simulink model "ctrl_clean_room_sim"  (R2015b)
settings: Solver=ode1  StartTime=0.0  StopTime=30  FixedStep=0.002  RelTol=1e-3
values from neighbouring files (symbols this model uses):
  K = place(A', C', p)'    [high_gain_pole_placement.m]    (also in tvlqr_feedback_trajectory.m = zeros(length(t), m, n); tvlqri_feedback_trajectory.m = zeros(length(t), m, n); weird_observer_pole_placement.m)
  lamb = [0  0  0  0  0; 0  0  0  0  0]    [dyn_ext_eps_static_meas.mat]    (also in extend_static_trajectory.m = repmat(lamb, samples, 1); high_gain_obs_test_meas_using_obs_for_contr.mat = [0 1.24633399283e-14 3.94751216865e-13 2.99125768707e-12 1.2; high_gain_obs_test_meas_using_obs_for_contr_2.mat = [0 0 0 0 0 0 0 0 0 0 0 0 ... (30000 elements, 6000x5)]; high_gain_obs_test_meas_using_obs_for_contr_3.mat = [0 0 0 0 0 0 0 0 0 0 0 0 ... (30000 elements, 6000x5)])
  logts = log.time    [ctr_sim_prepare_ws.m]
  logvals = zeros(numel(logts), n_signals)    [ctr_sim_prepare_ws.m]
  phi = [0  0  0; 0  0  0]    [dyn_ext_eps_static_meas.mat]    (also in extend_static_trajectory.m = repmat(phi, samples, 1); high_gain_obs_test_meas_using_obs_for_contr.mat = [1.104382406e-14 3.36532550257e-09 2.6875311489e-08 9.054493; high_gain_obs_test_meas_using_obs_for_contr_2.mat = [0 0 0 0 0 0 0 0 0 0 0 0 ... (18000 elements, 6000x3)]; high_gain_obs_test_meas_using_obs_for_contr_3.mat = [0 0 0 0 0 0 0 0 0 0 0 0 ... (18000 elements, 6000x3)])
  vb = [3.51031402612 3.51031402612]    [dyn_ext_eps_static_meas.mat]    (also in extend_static_trajectory.m = repmat(vb, samples, 1); high_gain_obs_test_meas_using_obs_for_contr.mat = [3.03305943788 3.03299005654 3.03292056635 3.03285098117 3.0; high_gain_obs_test_meas_using_obs_for_contr_2.mat = [2.46662433384 2.46662437608 2.46662467016 2.46662546356 2.4; high_gain_obs_test_meas_using_obs_for_contr_3.mat = [2.46662433384 2.46662437608 2.46662467016 2.46662546356 2.4)
  vf = [3.51031402612 3.51031402612]    [dyn_ext_eps_static_meas.mat]    (also in extend_static_trajectory.m = repmat(vf, samples, 1); high_gain_obs_test_meas_using_obs_for_contr.mat = [3.03305943788 3.03312882088 3.03319832259 3.03326793896 3.0; high_gain_obs_test_meas_using_obs_for_contr_2.mat = [2.46662433384 2.46662437608 2.46662467016 2.46662546356 2.4; high_gain_obs_test_meas_using_obs_for_contr_3.mat = [2.46662433384 2.46662437608 2.46662467016 2.46662546356 2.4)
undefined symbols (not defined in the file or in its folder): qc_get_step_size, R
libraries: simulink_extras x7, quarc_library x2, simulink x1
settings Model: Creator=Robert  LastModifiedBy=Robert

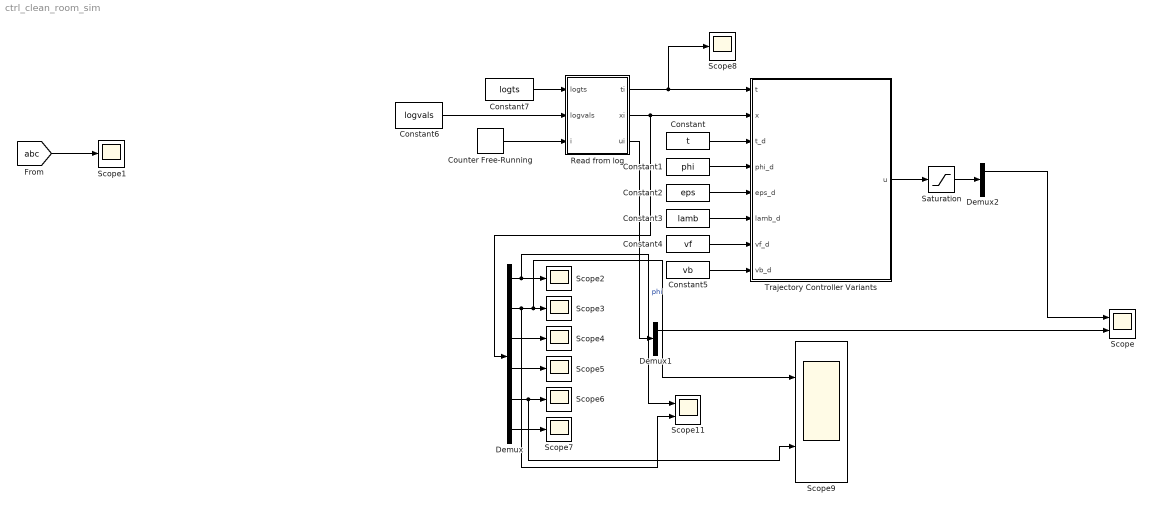
== system ctrl_clean_room_sim ==
  Constant : Constant  Value=t
  Constant1 : Constant  Value=phi
  Constant2 : Constant  Value=eps
  Constant3 : Constant  Value=lamb
  Constant4 : Constant  Value=vf
  Constant5 : Constant  Value=vb
  Constant6 : Constant  Value=logvals
  Constant7 : Constant  Value=logts
  Counter Free-Running : simulink/Sources/Counter Free-Running  NumBits=32  tsamp=-1
  Demux : Demux  Outputs=6
  Demux1 : Demux  Outputs=2
  Demux2 : Demux  Outputs=2
  Read from log : MATLAB Function  TreatAsAtomicUnit=on
  Saturation : Saturate  UpperLimit=5  LowerLimit=-5
  Scope : Scope  NumInputPorts=2
  Scope{1..8} (8 alike) : Scope
  Scope11 : Scope  NumInputPorts=2
  Scope9 : Scope  NumInputPorts=2
  Trajectory Controller Variants : Subsystem  Variant=on  OverrideUsingVariant=StateFeedback
  wires:
  Constant/1 -> Trajectory Controller Variants/3(t_d)
  Constant3/1 -> Trajectory Controller Variants/6(lamb_d)
  Constant2/1 -> Trajectory Controller Variants/5(eps_d)
  Constant1/1 -> Trajectory Controller Variants/4(phi_d)
  Constant5/1 -> Trajectory Controller Variants/8(vb_d)
  Constant4/1 -> Trajectory Controller Variants/7(vf_d)
  Read from log/2(xi) -> Demux/1, Trajectory Controller Variants/2(x)
  Read from log/1(ti) -> Scope8/1, Trajectory Controller Variants/1(t)
  Counter Free-Running/1 -> Read from log/3(i)
  Constant6/1 -> Read from log/2(logvals)
  Constant7/1 -> Read from log/1(logts)
  Read from log/3(ui) -> Demux1/1
  Trajectory Controller Variants/1(u) -> Saturation/1
  Saturation/1 -> Demux2/1
  Demux/1 -> Scope11/1, Scope2/1  "phi"
  Demux/2 -> Scope11/2, Scope9/1, Scope3/1
  Demux/3 -> Scope4/1
  Demux/4 -> Scope5/1
  Demux/5 -> Scope9/2, Scope6/1
  Demux/6 -> Scope7/1
  Demux2/1 -> Scope/1
  Demux1/1 -> Scope/2
  [abc] -> Scope1/1

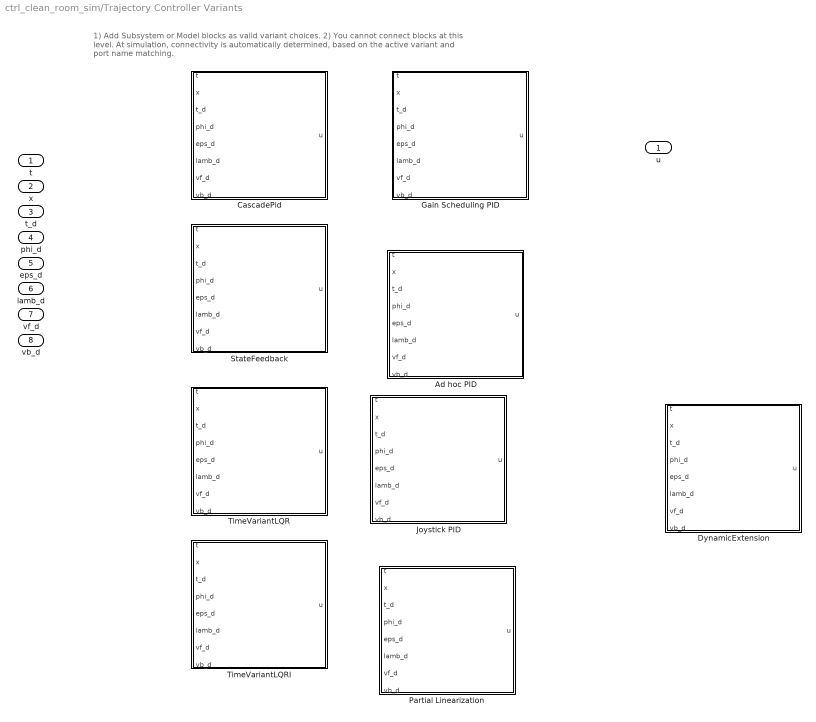
== system ctrl_clean_room_sim/Trajectory Controller Variants ==
  note: 1) Add Subsystem or Model blocks as valid variant choices.
      | 2) You cannot connect blocks at this level. At simulation, connectivity is automatically
      | determined, based on the active variant and port name matching.
  t : Inport
  x : Inport  Port=2  PortDimensions=6
  t_d : Inport  Port=3
  phi_d : Inport  Port=4
  eps_d : Inport  Port=5
  lamb_d : Inport  Port=6
  vf_d : Inport  Port=7
  vb_d : Inport  Port=8
  Ad hoc PID : Subsystem  VariantControl=AdHocPID
  CascadePid : Subsystem  VariantControl=CascadePid
  DynamicExtension : Subsystem  VariantControl=DynamicExtension
  Gain Scheduling PID : Subsystem  VariantControl=GainSchedulingPid
  Joystick PID : Subsystem  VariantControl=JoystickPID
  Partial Linearization : Subsystem  VariantControl=PartialLinearization
  StateFeedback : Subsystem  VariantControl=StateFeedback
  TimeVariantLQR : Subsystem  VariantControl=TimeVariantLQR
  TimeVariantLQRI : Subsystem  VariantControl=TimeVariantLQRI
  u : Outport

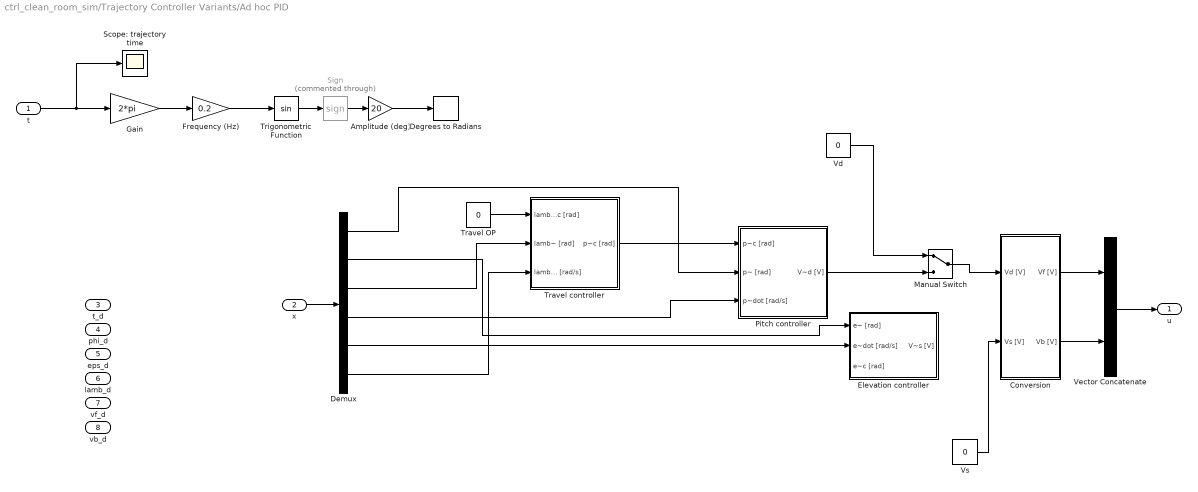
== system ctrl_clean_room_sim/Trajectory Controller Variants/Ad hoc PID ==
  t : Inport
  x : Inport  Port=2
  t_d : Inport  Port=3
  phi_d : Inport  Port=4
  eps_d : Inport  Port=5
  lamb_d : Inport  Port=6
  vf_d : Inport  Port=7
  vb_d : Inport  Port=8
  Amplitude (deg) : Gain  Gain=20
  Conversion : Subsystem
  Degrees to Radians : simulink_extras/Transformations/Degrees to Radians
  Demux : Demux  Outputs=6
  Elevation controller : Subsystem
  Frequency (Hz) : Gain  Gain=0.2
  Gain : Gain  Gain=2*pi
  Manual Switch : ManualSwitch
  Pitch controller : Subsystem
  Scope: trajectory time : Scope
  Sign : Signum  Commented=through
  Travel OP : Constant  Value=0
  Travel controller : Subsystem
  Trigonometric Function : Trigonometry
  Vd : Constant  Value=0
  Vector Concatenate : Concatenate
  Vs : Constant  Value=0
  u : Outport
  wires:
  Conversion/1(Vf [V]) -> Vector Concatenate/1
  Conversion/2(Vb [V]) -> Vector Concatenate/2
  x/1 -> Demux/1
  Demux/1 -> Pitch controller/2(p~ [rad])
  Demux/2 -> Elevation controller/1(e~ [rad])
  Demux/3 -> Travel controller/2(lamb~ [rad])
  Demux/4 -> Pitch controller/3(p~dot [rad/s])
  Demux/5 -> Elevation controller/2(e~dot [rad/s])
  Demux/6 -> Travel controller/3(lamb~dot [rad/s])
  Vector Concatenate/1 -> u/1
  t/1 -> Scope: trajectory time/1, Gain/1
  Gain/1 -> Frequency (Hz)/1
  Frequency (Hz)/1 -> Trigonometric Function/1
  Trigonometric Function/1 -> Sign/1
  Pitch controller/1(V~d [V]) -> Manual Switch/2
  Manual Switch/1 -> Conversion/1(Vd [V])
  Sign/1 -> Amplitude (deg)/1
  Amplitude (deg)/1 -> Degrees to Radians/1
  Travel controller/1(p~c [rad]) -> Pitch controller/1(p~c [rad])
  Travel OP/1 -> Travel controller/1(lamb~c [rad])
  Vd/1 -> Manual Switch/1
  Vs/1 -> Conversion/2(Vs [V])

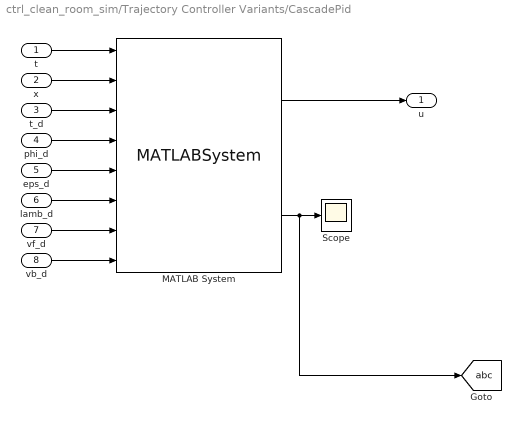
== system ctrl_clean_room_sim/Trajectory Controller Variants/CascadePid ==
  t : Inport
  x : Inport  Port=2
  t_d : Inport  Port=3
  phi_d : Inport  Port=4
  eps_d : Inport  Port=5
  lamb_d : Inport  Port=6
  vf_d : Inport  Port=7
  vb_d : Inport  Port=8
  MATLAB System : MATLABSystem  System=CascadePid  elevation_pid_gains=[15, 3, 7]  travel_pitch_pid_gains=[2.5, 0.5, 3]  pitch_vd_pid_gains=[4, 0.1, 2]  feed_forward=on  SimulateUsing=Code generation
      mask Type: CascadePid
      mask Display:
      | disp('CascadePid');
      | port_label('input',1,'Time');
      | port_label('input',2,'State');
      | port_label('input',3,'Traj Time');
      | port_label('input',4,'Traj Phi');
      | port_label('input',5,'Traj Eps');
      | port_label('input',6,'Traj Lamb');
      | port_label('input',7,'Traj Vf');
      | port_label('input',8,'Traj Vb');
      | port_label('output',1,'Control');
      | port_label('output',2,'Debug');
  Scope : Scope
  u : Outport
  tag scope: abc=global
  wires:
  MATLAB System/1 -> u/1
  vb_d/1 -> MATLAB System/8
  vf_d/1 -> MATLAB System/7
  lamb_d/1 -> MATLAB System/6
  eps_d/1 -> MATLAB System/5
  phi_d/1 -> MATLAB System/4
  t_d/1 -> MATLAB System/3
  x/1 -> MATLAB System/2
  t/1 -> MATLAB System/1
  MATLAB System/2 -> [abc], Scope/1

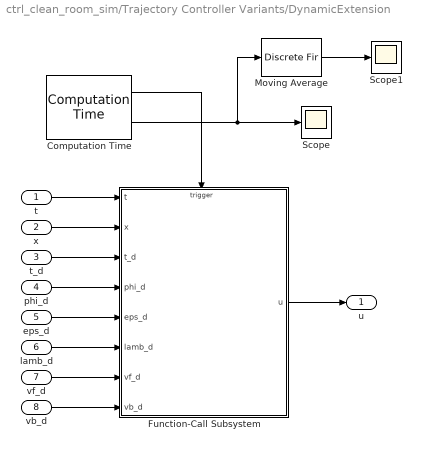
== system ctrl_clean_room_sim/Trajectory Controller Variants/DynamicExtension ==
  t : Inport
  x : Inport  Port=2
  t_d : Inport  Port=3
  phi_d : Inport  Port=4
  eps_d : Inport  Port=5
  lamb_d : Inport  Port=6
  vf_d : Inport  Port=7
  vb_d : Inport  Port=8
  Computation Time : quarc_library/Sources/Time/Computation Time  sample_time=qc_get_step_size  use_model=off
  Function-Call Subsystem : Subsystem  TreatAsAtomicUnit=on
  Moving Average : DiscreteFir  Coefficients=ones(1, 50) / 50
  Scope : Scope
  Scope1 : Scope
  u : Outport
  wires:
  vb_d/1 -> Function-Call Subsystem/8(vb_d)
  vf_d/1 -> Function-Call Subsystem/7(vf_d)
  lamb_d/1 -> Function-Call Subsystem/6(lamb_d)
  eps_d/1 -> Function-Call Subsystem/5(eps_d)
  phi_d/1 -> Function-Call Subsystem/4(phi_d)
  t_d/1 -> Function-Call Subsystem/3(t_d)
  x/1 -> Function-Call Subsystem/2(x)
  t/1 -> Function-Call Subsystem/1(t)
  Function-Call Subsystem/1(u) -> u/1
  Computation Time/1 -> Function-Call Subsystem/Trigger
  Computation Time/2 -> Moving Average/1, Scope/1
  Moving Average/1 -> Scope1/1

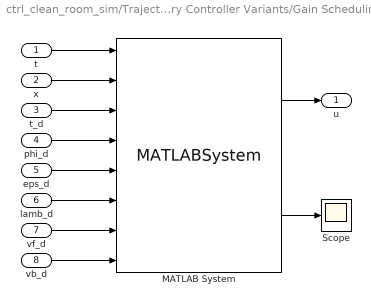
== system ctrl_clean_room_sim/Trajectory Controller Variants/Gain Scheduling PID ==
  t : Inport
  x : Inport  Port=2
  t_d : Inport  Port=3
  phi_d : Inport  Port=4
  eps_d : Inport  Port=5
  lamb_d : Inport  Port=6
  vf_d : Inport  Port=7
  vb_d : Inport  Port=8
  MATLAB System : MATLABSystem  System=GainSchedulingPid  elevation_levels=[ -10, 0, 10, 20 ]  elevation_pid_gains=[15, 3, 7]  travel_pitch_pid_gains=[2.5, 0.1, 3.2; 4, 0.1, 3.5; 4, 0.1, 3.25; 2.5, 0.1, 2.5]  pitch_vd_pid_gains=[ 4, 0.1, 2 ]  feed_forward=on  SimulateUsing=Code generation
      mask Type: GainSchedulingPid
      mask Display:
      | disp('GainSchedulingPid');
      | port_label('input',1,'Time');
      | port_label('input',2,'State');
      | port_label('input',3,'Traj Time');
      | port_label('input',4,'Traj Phi');
      | port_label('input',5,'Traj Eps');
      | port_label('input',6,'Traj Lamb');
      | port_label('input',7,'Traj Vf');
      | port_label('input',8,'Traj Vb');
      | port_label('output',1,'Control');
      | port_label('output',2,'Debug');
  Scope : Scope
  u : Outport
  wires:
  MATLAB System/1 -> u/1
  vb_d/1 -> MATLAB System/8
  vf_d/1 -> MATLAB System/7
  lamb_d/1 -> MATLAB System/6
  eps_d/1 -> MATLAB System/5
  phi_d/1 -> MATLAB System/4
  t_d/1 -> MATLAB System/3
  x/1 -> MATLAB System/2
  t/1 -> MATLAB System/1
  MATLAB System/2 -> Scope/1

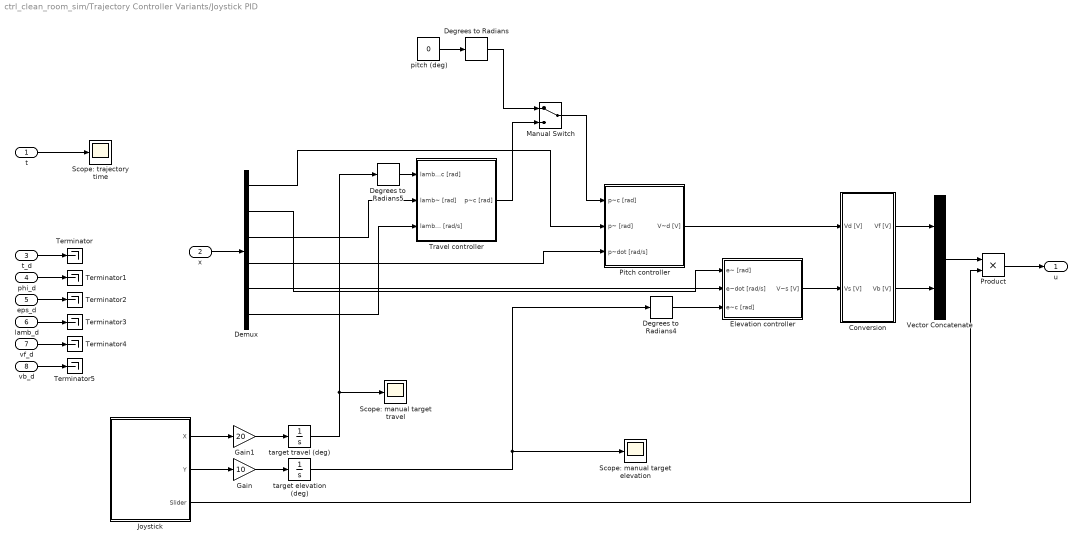
== system ctrl_clean_room_sim/Trajectory Controller Variants/Joystick PID ==
  t : Inport
  x : Inport  Port=2
  t_d : Inport  Port=3
  phi_d : Inport  Port=4
  eps_d : Inport  Port=5
  lamb_d : Inport  Port=6
  vf_d : Inport  Port=7
  vb_d : Inport  Port=8
  Conversion : Subsystem
  Degrees to Radians : simulink_extras/Transformations/Degrees to Radians
  Degrees to Radians4 : simulink_extras/Transformations/Degrees to Radians
  Degrees to Radians5 : simulink_extras/Transformations/Degrees to Radians
  Demux : Demux  Outputs=6
  Elevation controller : Subsystem
  Gain : Gain  Gain=10
  Gain1 : Gain  Gain=20
  Joystick : Subsystem
  Manual Switch : ManualSwitch
  Pitch controller : Subsystem
  Product : Product
  Scope: manual target elevation : Scope
  Scope: manual target travel : Scope
  Scope: trajectory time : Scope
  Terminator{,1..5} (6 alike) : Terminator
  Travel controller : Subsystem
  Vector Concatenate : Concatenate
  pitch (deg) : Constant  Value=0
  target elevation (deg) : Integrator  InitialCondition=-29  LimitOutput=on  UpperSaturationLimit=30  LowerSaturationLimit=-30
  target travel (deg) : Integrator  LimitOutput=on  UpperSaturationLimit=180  LowerSaturationLimit=-180
  u : Outport
  wires:
  Conversion/1(Vf [V]) -> Vector Concatenate/1
  Conversion/2(Vb [V]) -> Vector Concatenate/2
  Elevation controller/1(V~s [V]) -> Conversion/2(Vs [V])
  Pitch controller/1(V~d [V]) -> Conversion/1(Vd [V])
  x/1 -> Demux/1
  Demux/1 -> Pitch controller/2(p~ [rad])
  Demux/2 -> Elevation controller/1(e~ [rad])
  Demux/3 -> Travel controller/2(lamb~ [rad])
  Demux/4 -> Pitch controller/3(p~dot [rad/s])
  Demux/5 -> Elevation controller/2(e~dot [rad/s])
  Demux/6 -> Travel controller/3(lamb~dot [rad/s])
  Degrees to Radians5/1 -> Travel controller/1(lamb~c [rad])
  Degrees to Radians4/1 -> Elevation controller/3(e~c [rad])
  Joystick/2(Y) -> Gain/1
  Gain/1 -> target elevation (deg)/1
  Joystick/1(X) -> Gain1/1
  Gain1/1 -> target travel (deg)/1
  target elevation (deg)/1 -> Scope: manual target elevation/1, Degrees to Radians4/1
  target travel (deg)/1 -> Scope: manual target travel/1, Degrees to Radians5/1
  Vector Concatenate/1 -> Product/1
  Product/1 -> u/1
  Joystick/3(Slider) -> Product/2
  t/1 -> Scope: trajectory time/1
  Manual Switch/1 -> Pitch controller/1(p~c [rad])
  Travel controller/1(p~c [rad]) -> Manual Switch/2
  pitch (deg)/1 -> Degrees to Radians/1
  Degrees to Radians/1 -> Manual Switch/1
  t_d/1 -> Terminator/1
  phi_d/1 -> Terminator1/1
  eps_d/1 -> Terminator2/1
  lamb_d/1 -> Terminator3/1
  vf_d/1 -> Terminator4/1
  vb_d/1 -> Terminator5/1

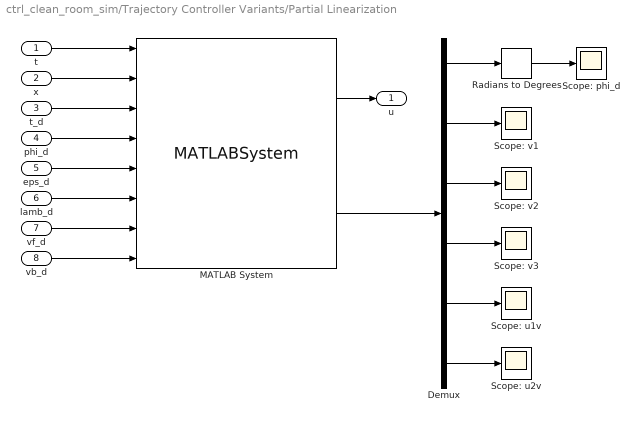
== system ctrl_clean_room_sim/Trajectory Controller Variants/Partial Linearization ==
  t : Inport
  x : Inport  Port=2
  t_d : Inport  Port=3
  phi_d : Inport  Port=4
  eps_d : Inport  Port=5
  lamb_d : Inport  Port=6
  vf_d : Inport  Port=7
  vb_d : Inport  Port=8
  Demux : Demux  Outputs=6
  MATLAB System : MATLABSystem  System=FeedbackLinearization  ke=[ 6, 3 ]  kl=[3, 4]  kp=[ 40, 20 ]  SimulateUsing=Code generation
      mask Type: FeedbackLinearization
      mask Display:
      | disp('FeedbackLinearization');
      | port_label('input',1,'Time');
      | port_label('input',2,'State');
      | port_label('input',3,'Traj Time');
      | port_label('input',4,'Traj Phi');
      | port_label('input',5,'Traj Eps');
      | port_label('input',6,'Traj Lamb');
      | port_label('input',7,'Traj Vf');
      | port_label('input',8,'Traj Vb');
      | port_label('output',1,'Control');
      | port_label('output',2,'Debug');
  Radians to Degrees : simulink_extras/Transformations/Radians to Degrees
  Scope: phi_d : Scope
  Scope: u1v : Scope
  Scope: u2v : Scope
  Scope: v1 : Scope
  Scope: v2 : Scope
  Scope: v3 : Scope
  u : Outport
  wires:
  MATLAB System/1 -> u/1
  vb_d/1 -> MATLAB System/8
  vf_d/1 -> MATLAB System/7
  lamb_d/1 -> MATLAB System/6
  eps_d/1 -> MATLAB System/5
  phi_d/1 -> MATLAB System/4
  t_d/1 -> MATLAB System/3
  x/1 -> MATLAB System/2
  t/1 -> MATLAB System/1
  MATLAB System/2 -> Demux/1
  Demux/1 -> Radians to Degrees/1
  Radians to Degrees/1 -> Scope: phi_d/1
  Demux/2 -> Scope: v1/1
  Demux/3 -> Scope: v2/1
  Demux/4 -> Scope: v3/1
  Demux/5 -> Scope: u1v/1
  Demux/6 -> Scope: u2v/1

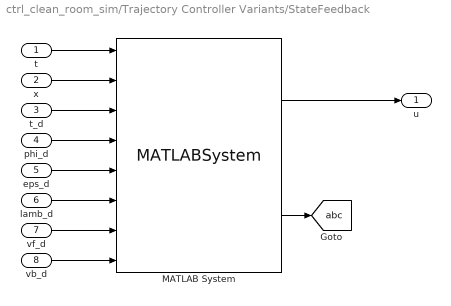
== system ctrl_clean_room_sim/Trajectory Controller Variants/StateFeedback ==
  t : Inport
  x : Inport  Port=2
  t_d : Inport  Port=3
  phi_d : Inport  Port=4
  eps_d : Inport  Port=5
  lamb_d : Inport  Port=6
  vf_d : Inport  Port=7
  vb_d : Inport  Port=8
  MATLAB System : MATLABSystem  System=StateFeedback  K=K  SimulateUsing=Code generation
      mask Type: StateFeedback
      mask Display:
      | disp('StateFeedback');
      | port_label('input',1,'Time');
      | port_label('input',2,'State');
      | port_label('input',3,'Traj Time');
      | port_label('input',4,'Traj Phi');
      | port_label('input',5,'Traj Eps');
      | port_label('input',6,'Traj Lamb');
      | port_label('input',7,'Traj Vf');
      | port_label('input',8,'Traj Vb');
      | port_label('output',1,'Control');
      | port_label('output',2,'Debug');
  u : Outport
  tag scope: abc=global
  wires:
  MATLAB System/1 -> u/1
  vb_d/1 -> MATLAB System/8
  vf_d/1 -> MATLAB System/7
  lamb_d/1 -> MATLAB System/6
  eps_d/1 -> MATLAB System/5
  phi_d/1 -> MATLAB System/4
  t_d/1 -> MATLAB System/3
  x/1 -> MATLAB System/2
  t/1 -> MATLAB System/1
  MATLAB System/2 -> [abc]

== system ctrl_clean_room_sim/Trajectory Controller Variants/TimeVariantLQR ==
  t : Inport
  x : Inport  Port=2
  t_d : Inport  Port=3
  phi_d : Inport  Port=4
  eps_d : Inport  Port=5
  lamb_d : Inport  Port=6
  vf_d : Inport  Port=7
  vb_d : Inport  Port=8
  MATLAB System : MATLABSystem  System=TimeVariantLQR  Q=Q  R=R  S=S  riccati_tau=riccati_tau  riccati_P_triu_tau=riccati_P_triu_tau  SimulateUsing=Code generation
      mask Type: TimeVariantLQR
      mask Display:
      | disp('TimeVariantLQR');
      | port_label('input',1,'Time');
      | port_label('input',2,'State');
      | port_label('input',3,'Traj Time');
      | port_label('input',4,'Traj Phi');
      | port_label('input',5,'Traj Eps');
      | port_label('input',6,'Traj Lamb');
      | port_label('input',7,'Traj Vf');
      | port_label('input',8,'Traj Vb');
      | port_label('output',1,'Control');
      | port_label('output',2,'Debug');
  u : Outport
  wires:
  MATLAB System/1 -> u/1
  vb_d/1 -> MATLAB System/8
  vf_d/1 -> MATLAB System/7
  lamb_d/1 -> MATLAB System/6
  eps_d/1 -> MATLAB System/5
  phi_d/1 -> MATLAB System/4
  t_d/1 -> MATLAB System/3
  x/1 -> MATLAB System/2
  t/1 -> MATLAB System/1

== system ctrl_clean_room_sim/Trajectory Controller Variants/TimeVariantLQRI ==
  t : Inport
  x : Inport  Port=2
  t_d : Inport  Port=3
  phi_d : Inport  Port=4
  eps_d : Inport  Port=5
  lamb_d : Inport  Port=6
  vf_d : Inport  Port=7
  vb_d : Inport  Port=8
  MATLAB System : MATLABSystem  System=TimeVariantLQRI  Q=Q  R=R  S=S  riccati_tau=riccati_tau  riccati_P_triu_tau=riccati_P_triu_tau  step_width=0.002  SimulateUsing=Code generation
      mask Type: TimeVariantLQRI
      mask Display:
      | disp('TimeVariantLQRI');
      | port_label('input',1,'Time');
      | port_label('input',2,'State');
      | port_label('input',3,'Traj Time');
      | port_label('input',4,'Traj Phi');
      | port_label('input',5,'Traj Eps');
      | port_label('input',6,'Traj Lamb');
      | port_label('input',7,'Traj Vf');
      | port_label('input',8,'Traj Vb');
      | port_label('output',1,'Control');
      | port_label('output',2,'Debug');
  u : Outport
  wires:
  MATLAB System/1 -> u/1
  vb_d/1 -> MATLAB System/8
  vf_d/1 -> MATLAB System/7
  lamb_d/1 -> MATLAB System/6
  eps_d/1 -> MATLAB System/5
  phi_d/1 -> MATLAB System/4
  t_d/1 -> MATLAB System/3
  x/1 -> MATLAB System/2
  t/1 -> MATLAB System/1

== system ctrl_clean_room_sim/Trajectory Controller Variants/Ad hoc PID/Conversion ==
  Vd [V] : Inport
  Vs [V] : Inport  Port=2
  Add : Sum
  Back gain : Gain  Gain=0.5
  Front gain : Gain  Gain=0.5
  Subtract : Sum  Inputs=+-
  Vf [V] : Outport
  Vb [V] : Outport  Port=2
  wires:
  Vd [V]/1 -> Subtract/2, Add/1
  Vs [V]/1 -> Subtract/1, Add/2
  Subtract/1 -> Back gain/1
  Back gain/1 -> Vb [V]/1
  Add/1 -> Front gain/1
  Front gain/1 -> Vf [V]/1

== system ctrl_clean_room_sim/Trajectory Controller Variants/Ad hoc PID/Elevation controller ==
  e~ [rad] : Inport
  e~dot [rad/s] : Inport  Port=2
  e~c [rad] : Inport  Port=3
  Elevation controller : Subsystem
  Sum : Sum  Inputs=-+  SaturateOnIntegerOverflow=on  InputSameDT=on  OutDataTypeStr=Inherit: Same as first input
  V~s [V] : Outport  InitialOutput=0
  wires:
  Sum/1 -> Elevation controller/1(e~ [rad])
  Elevation controller/1(V~_s [V]) -> V~s [V]/1
  e~ [rad]/1 -> Sum/1
  e~dot [rad/s]/1 -> Elevation controller/2(e~_dot [rad/s])
  e~c [rad]/1 -> Sum/2

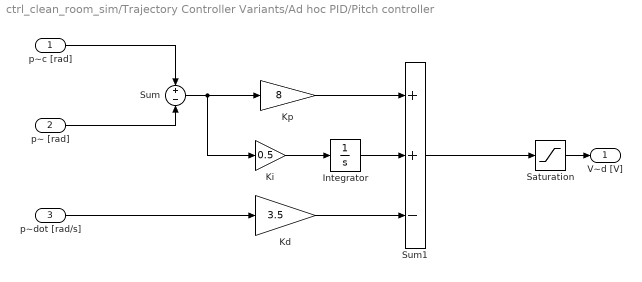
== system ctrl_clean_room_sim/Trajectory Controller Variants/Ad hoc PID/Pitch controller ==
  p~c [rad] : Inport
  p~ [rad] : Inport  Port=2
  p~dot [rad/s] : Inport  Port=3
  Integrator : Integrator  LimitOutput=on
  Kd : Gain  Gain=3.5
  Ki : Gain  Gain=0.5
  Kp : Gain  Gain=8
  Saturation : Saturate  UpperLimit=10  LowerLimit=-10
  Sum : Sum  Inputs=+-
  Sum1 : Sum  Inputs=++-
  V~d [V] : Outport  InitialOutput=0
  wires:
  p~c [rad]/1 -> Sum/1
  p~ [rad]/1 -> Sum/2
  Sum/1 -> Ki/1, Kp/1
  p~dot [rad/s]/1 -> Kd/1
  Kp/1 -> Sum1/1
  Sum1/1 -> Saturation/1
  Saturation/1 -> V~d [V]/1
  Kd/1 -> Sum1/3
  Ki/1 -> Integrator/1
  Integrator/1 -> Sum1/2

== system ctrl_clean_room_sim/Trajectory Controller Variants/Ad hoc PID/Travel controller ==
  lamb~c [rad] : Inport
  lamb~ [rad] : Inport  Port=2
  lamb~dot [rad/s] : Inport  Port=3
  Integrator : Integrator  LimitOutput=on  UpperSaturationLimit=45/180*pi  LowerSaturationLimit=-45/180*pi
  Kd : Gain  Gain=1.2
  Ki : Gain  Gain=0.02
  Kp : Gain  Gain=0.7
  Saturation : Saturate  UpperLimit=45/180*pi  LowerLimit=-45/180*pi
  Sum : Sum  Inputs=+-
  Sum1 : Sum  Inputs=++-
  p~c [rad] : Outport  InitialOutput=0
  wires:
  lamb~c [rad]/1 -> Sum/1
  lamb~ [rad]/1 -> Sum/2
  Sum/1 -> Ki/1, Kp/1
  lamb~dot [rad/s]/1 -> Kd/1
  Kp/1 -> Sum1/1
  Saturation/1 -> p~c [rad]/1
  Kd/1 -> Sum1/3
  Ki/1 -> Integrator/1
  Integrator/1 -> Sum1/2
  Sum1/1 -> Saturation/1

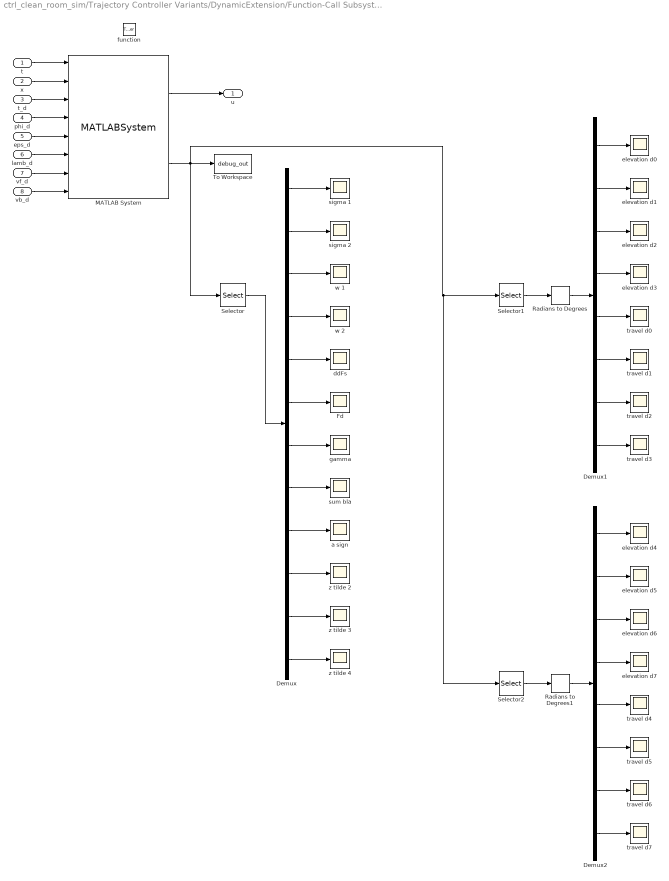
== system ctrl_clean_room_sim/Trajectory Controller Variants/DynamicExtension/Function-Call Subsystem ==
  t : Inport
  x : Inport  Port=2
  t_d : Inport  Port=3
  phi_d : Inport  Port=4
  eps_d : Inport  Port=5
  lamb_d : Inport  Port=6
  vf_d : Inport  Port=7
  vb_d : Inport  Port=8
  function : TriggerPort  TriggerType=function-call
  Demux : Demux  Outputs=12
  Demux1 : Demux  Outputs=8
  Demux2 : Demux  Outputs=8
  Fd : Scope
  MATLAB System : MATLABSystem  System=DynamicExtension  k_eps=[256 256 96 16]  k_lamb=[170 133.5 66.25 23]  a1=20  a2=30  b1=100  b2=0.1  K=[5.78137039154897e-17 8.03194586412948 7.37873334683116e-15 -1.60527626610439 0.496517662944292;-8.37957307173646e-13 13.583071210233 -9.11470856007611e-14 -5.11296015147329 1.98832652424711;6.17959795944787e-13 -11.5048935665947 8.9697895932897e-14 5.73851966383715 0.161103489630765;1.00112915950762e-12 -18.6946906139968 1.59587847685695e-13 7.45245581619715 1.38532374485326;-0.0478278821751323 -1.15484672098923e-14 5.69499260004304 4.71520176801062e-14 4.19145017494709e-14;0.901038014382726 -2.42942309534905e-14 6.28853856730032 7.08845076170615e-14 9.52974747824829e-14;4.94324192305077 -6.93413110170475e-13 -1.98914667214254 1.29306967899618e-12 -2.66124009261711e-13;5.89970873116958 -2.02737451517472e-12 0.427493186857978 3.23952773786289e-12 -5.5159720578489e-13]  x780=x780  z_est0=z_est0  x_est0=x_est0  step_width=0.002  smc=off  use_high_gain_observer=off  use_weird_observer=off  SimulateUsing=Code generation
      mask Type: DynamicExtension
      mask Display:
      | disp('DynamicExtension');
      | port_label('input',1,'Time');
      | port_label('input',2,'State');
      | port_label('input',3,'Traj Time');
      | port_label('input',4,'Traj Phi');
      | port_label('input',5,'Traj Eps');
      | port_label('input',6,'Traj Lamb');
      | port_label('input',7,'Traj Vf');
      | port_label('input',8,'Traj Vb');
      | port_label('output',1,'Control');
      | port_label('output',2,'Debug');
  Radians to Degrees : simulink_extras/Transformations/Radians to Degrees
  Radians to Degrees1 : simulink_extras/Transformations/Radians to Degrees
  Selector : Selector  InputPortWidth=44  IndexOptions=Index vector (dialog)  Indices=25:36  OutputSizes=1
  Selector1 : Selector  InputPortWidth=44  IndexOptions=Index vector (dialog)  Indices=37:44  OutputSizes=1
  Selector2 : Selector  InputPortWidth=44  IndexOptions=Index vector (dialog)  Indices=17:24  OutputSizes=1
  To Workspace : ToWorkspace  VariableName=debug_out  SaveFormat=Structure With Time  SampleTime=-1
  a sign : Scope
  ddFs : Scope
  elevation d{0..7} (8 alike) : Scope
  gamma : Scope
  sigma 1 : Scope
  sigma 2 : Scope
  sum bla : Scope
  travel d{0..7} (8 alike) : Scope
  w 1 : Scope
  w 2 : Scope
  z tilde 2 : Scope
  z tilde 3 : Scope
  z tilde 4 : Scope
  u : Outport
  wires:
  vb_d/1 -> MATLAB System/8
  vf_d/1 -> MATLAB System/7
  lamb_d/1 -> MATLAB System/6
  eps_d/1 -> MATLAB System/5
  phi_d/1 -> MATLAB System/4
  t_d/1 -> MATLAB System/3
  x/1 -> MATLAB System/2
  t/1 -> MATLAB System/1
  MATLAB System/1 -> u/1
  MATLAB System/2 -> Selector2/1, Selector1/1, Selector/1, To Workspace/1
  Selector/1 -> Demux/1
  Demux/1 -> sigma 1/1
  Demux/2 -> sigma 2/1
  Demux/3 -> w 1/1
  Demux/4 -> w 2/1
  Demux/5 -> ddFs/1
  Demux/6 -> Fd/1
  Demux/7 -> gamma/1
  Demux/8 -> sum bla/1
  Demux/9 -> a sign/1
  Demux/10 -> z tilde 2/1
  Demux/11 -> z tilde 3/1
  Demux/12 -> z tilde 4/1
  Selector1/1 -> Radians to Degrees/1
  Demux1/1 -> elevation d0/1
  Demux1/2 -> elevation d1/1
  Demux1/3 -> elevation d2/1
  Demux1/4 -> elevation d3/1
  Demux1/5 -> travel d0/1
  Demux1/6 -> travel d1/1
  Demux1/7 -> travel d2/1
  Demux1/8 -> travel d3/1
  Radians to Degrees/1 -> Demux1/1
  Selector2/1 -> Radians to Degrees1/1
  Demux2/1 -> elevation d4/1
  Demux2/2 -> elevation d5/1
  Demux2/3 -> elevation d6/1
  Demux2/4 -> elevation d7/1
  Demux2/5 -> travel d4/1
  Demux2/6 -> travel d5/1
  Demux2/7 -> travel d6/1
  Demux2/8 -> travel d7/1
  Radians to Degrees1/1 -> Demux2/1

== system ctrl_clean_room_sim/Trajectory Controller Variants/Joystick PID/Conversion ==
  Vd [V] : Inport
  Vs [V] : Inport  Port=2
  Add : Sum
  Back gain : Gain  Gain=0.5
  Front gain : Gain  Gain=0.5
  Subtract : Sum  Inputs=+-
  Vf [V] : Outport
  Vb [V] : Outport  Port=2
  wires:
  Vd [V]/1 -> Subtract/2, Add/1
  Vs [V]/1 -> Subtract/1, Add/2
  Subtract/1 -> Back gain/1
  Back gain/1 -> Vb [V]/1
  Add/1 -> Front gain/1
  Front gain/1 -> Vf [V]/1

== system ctrl_clean_room_sim/Trajectory Controller Variants/Joystick PID/Elevation controller ==
  e~ [rad] : Inport
  e~dot [rad/s] : Inport  Port=2
  e~c [rad] : Inport  Port=3
  Elevation controller : Subsystem
  Sum : Sum  Inputs=-+  SaturateOnIntegerOverflow=on  InputSameDT=on  OutDataTypeStr=Inherit: Same as first input
  V~s [V] : Outport  InitialOutput=0
  wires:
  Sum/1 -> Elevation controller/1(e~ [rad])
  Elevation controller/1(V~_s [V]) -> V~s [V]/1
  e~ [rad]/1 -> Sum/1
  e~dot [rad/s]/1 -> Elevation controller/2(e~_dot [rad/s])
  e~c [rad]/1 -> Sum/2

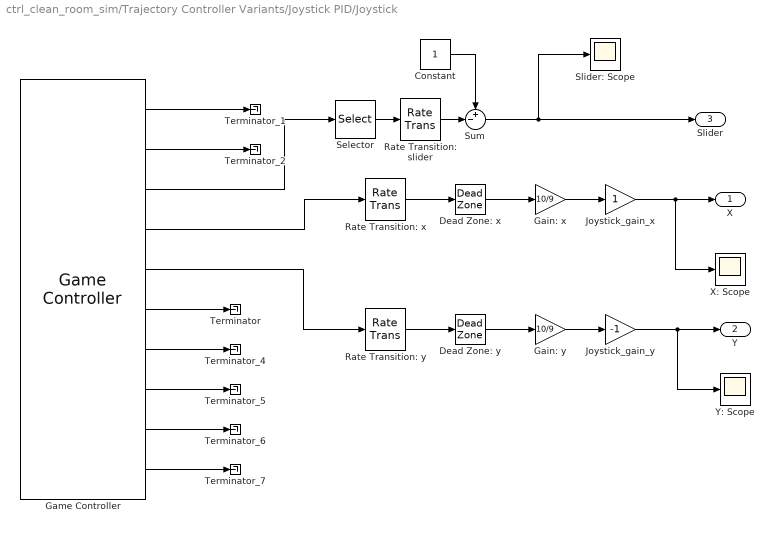
== system ctrl_clean_room_sim/Trajectory Controller Variants/Joystick PID/Joystick ==
  Constant : Constant
  Dead Zone: x : DeadZone  LowerValue=-0.1  UpperValue=0.1  SaturateOnIntegerOverflow=on
  Dead Zone: y : DeadZone  LowerValue=-0.1  UpperValue=0.1  SaturateOnIntegerOverflow=on
  Gain: x : Gain  Gain=10/9
  Gain: y : Gain  Gain=10/9
  Game Controller : quarc_library/Devices/Peripherals/Target/Game Controller  controller=1  buffer_size=12  deadzone=[]  saturation=[]  sample_time=max(qc_get_step_size, 0.01)  auto_center=off  enabled=on
  Joystick_gain_x : Gain
  Joystick_gain_y : Gain  Gain=-1
  Rate Transition: slider : RateTransition
  Rate Transition: x : RateTransition
  Rate Transition: y : RateTransition
  Selector : Selector  InputPortWidth=2  IndexOptions=Index vector (dialog)  Indices=1  OutputSizes=1
  Slider: Scope : Scope
  Sum : Sum  Inputs=+-|
  Terminator : Terminator
  Terminator_{1..2,4..7} (6 alike) : Terminator
  X: Scope : Scope
  Y: Scope : Scope
  X : Outport
  Y : Outport  Port=2
  Slider : Outport  Port=3
  wires:
  Rate Transition: y/1 -> Dead Zone: y/1
  Rate Transition: x/1 -> Dead Zone: x/1
  Game Controller/5 -> Rate Transition: y/1
  Game Controller/4 -> Rate Transition: x/1
  Game Controller/1 -> Terminator_1/1
  Game Controller/2 -> Terminator_2/1
  Game Controller/7 -> Terminator_4/1
  Game Controller/8 -> Terminator_5/1
  Game Controller/9 -> Terminator_6/1
  Game Controller/10 -> Terminator_7/1
  Game Controller/3 -> Selector/1
  Game Controller/6 -> Terminator/1
  Dead Zone: x/1 -> Gain: x/1
  Dead Zone: y/1 -> Gain: y/1
  Gain: x/1 -> Joystick_gain_x/1
  Gain: y/1 -> Joystick_gain_y/1
  Joystick_gain_x/1 -> X/1, X: Scope/1
  Joystick_gain_y/1 -> Y: Scope/1, Y/1
  Sum/1 -> Slider/1, Slider: Scope/1
  Constant/1 -> Sum/1
  Selector/1 -> Rate Transition: slider/1
  Rate Transition: slider/1 -> Sum/2

== system ctrl_clean_room_sim/Trajectory Controller Variants/Joystick PID/Pitch controller ==
  p~c [rad] : Inport
  p~ [rad] : Inport  Port=2
  p~dot [rad/s] : Inport  Port=3
  Integrator : Integrator  LimitOutput=on
  Kd : Gain  Gain=3.5
  Ki : Gain  Gain=0.5
  Kp : Gain  Gain=8
  Saturation : Saturate  UpperLimit=10  LowerLimit=-10
  Sum : Sum  Inputs=+-
  Sum1 : Sum  Inputs=++-
  V~d [V] : Outport  InitialOutput=0
  wires:
  p~c [rad]/1 -> Sum/1
  p~ [rad]/1 -> Sum/2
  Sum/1 -> Ki/1, Kp/1
  p~dot [rad/s]/1 -> Kd/1
  Kp/1 -> Sum1/1
  Sum1/1 -> Saturation/1
  Saturation/1 -> V~d [V]/1
  Kd/1 -> Sum1/3
  Ki/1 -> Integrator/1
  Integrator/1 -> Sum1/2

== system ctrl_clean_room_sim/Trajectory Controller Variants/Joystick PID/Travel controller ==
  lamb~c [rad] : Inport
  lamb~ [rad] : Inport  Port=2
  lamb~dot [rad/s] : Inport  Port=3
  Integrator : Integrator  LimitOutput=on
  Kd : Gain  Gain=1.8
  Ki : Gain  Gain=0.005
  Kp : Gain  Gain=1.5
  Saturation : Saturate  UpperLimit=20  LowerLimit=-20
  Sum : Sum  Inputs=+-
  Sum1 : Sum  Inputs=++-
  p~c [rad] : Outport  InitialOutput=0
  wires:
  lamb~c [rad]/1 -> Sum/1
  lamb~ [rad]/1 -> Sum/2
  Sum/1 -> Ki/1, Kp/1
  lamb~dot [rad/s]/1 -> Kd/1
  Kp/1 -> Sum1/1
  Saturation/1 -> p~c [rad]/1
  Kd/1 -> Sum1/3
  Ki/1 -> Integrator/1
  Integrator/1 -> Sum1/2
  Sum1/1 -> Saturation/1

== system ctrl_clean_room_sim/Trajectory Controller Variants/Ad hoc PID/Elevation controller/Elevation controller ==
  e~ [rad] : Inport
  e~_dot [rad/s] : Inport  Port=2
  Integrator : Integrator  LimitOutput=on
  K_ed : Gain  Gain=20  SaturateOnIntegerOverflow=on  OutDataTypeStr=Inherit: Same as input  ParamDataTypeStr=Inherit: Same as input
  K_ei : Gain  Gain=20  SaturateOnIntegerOverflow=on  OutDataTypeStr=Inherit: Same as input  ParamDataTypeStr=Inherit: Same as input
  K_ep : Gain  Gain=30  SaturateOnIntegerOverflow=on  OutDataTypeStr=Inherit: Same as input  ParamDataTypeStr=Inherit: Same as input
  Sum : Sum  Inputs=++-  SaturateOnIntegerOverflow=on  InputSameDT=on  OutDataTypeStr=Inherit: Same as first input
  V~_s [V] : Outport  InitialOutput=0
  wires:
  K_ei/1 -> Integrator/1
  Integrator/1 -> Sum/1
  Sum/1 -> V~_s [V]/1
  e~_dot [rad/s]/1 -> K_ed/1
  K_ed/1 -> Sum/3
  K_ep/1 -> Sum/2
  e~ [rad]/1 -> K_ep/1, K_ei/1

== system ctrl_clean_room_sim/Trajectory Controller Variants/Joystick PID/Elevation controller/Elevation controller ==
  e~ [rad] : Inport
  e~_dot [rad/s] : Inport  Port=2
  Integrator : Integrator  LimitOutput=on
  K_ed : Gain  Gain=12  SaturateOnIntegerOverflow=on  OutDataTypeStr=Inherit: Same as input  ParamDataTypeStr=Inherit: Same as input
  K_ei : Gain  Gain=5  SaturateOnIntegerOverflow=on  OutDataTypeStr=Inherit: Same as input  ParamDataTypeStr=Inherit: Same as input
  K_ep : Gain  Gain=15  SaturateOnIntegerOverflow=on  OutDataTypeStr=Inherit: Same as input  ParamDataTypeStr=Inherit: Same as input
  Sum : Sum  Inputs=++-  SaturateOnIntegerOverflow=on  InputSameDT=on  OutDataTypeStr=Inherit: Same as first input
  V~_s [V] : Outport  InitialOutput=0
  wires:
  K_ei/1 -> Integrator/1
  Integrator/1 -> Sum/1
  Sum/1 -> V~_s [V]/1
  e~_dot [rad/s]/1 -> K_ed/1
  K_ed/1 -> Sum/3
  K_ep/1 -> Sum/2
  e~ [rad]/1 -> K_ep/1, K_ei/1

== matlab function ctrl_clean_room_sim/Read from log ==
  data: logts input; logvals input; ti output size=1; xi output; i input; ui output
function [ti, xi, ui] = fcn(logts, logvals, i)
enable_ramping = logvals(:, 6);
start_index = find(enable_ramping == -1, 1);
start_index = start_index(1);

i = start_index+i;

ti = logts(i) - logts(start_index);
xi = logvals(i, 7:12)';
ui = logvals(i, 1:2)';
